simulink model "SinglePhaseControlledConveter"  (R2024a)
settings: Solver=VariableStepAuto  StartTime=0.0  StopTime=0.1  RelTol=1e-3
libraries: spsThyristorLib x4, spsCurrentMeasurementLib x2, spsVoltageMeasurementLib x2, spsACVoltageSourceLib x1, spsGroundLib x1, spsSeriesRLCBranchLib x1, spspowerguiLib x1
settings Model: Creator=danielmcguiness  LastModifiedBy=danielmcguiness

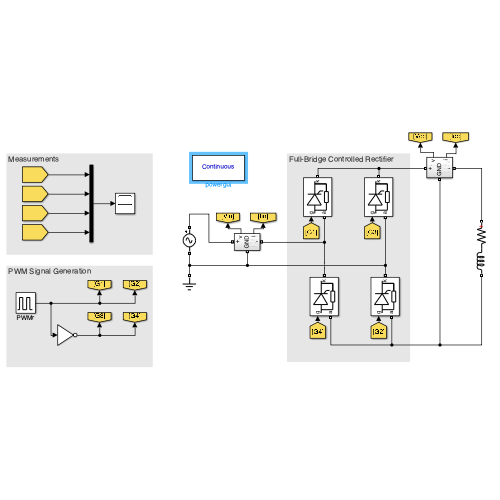
[thumbnail: Simulink's stored preview of the top-level diagram]
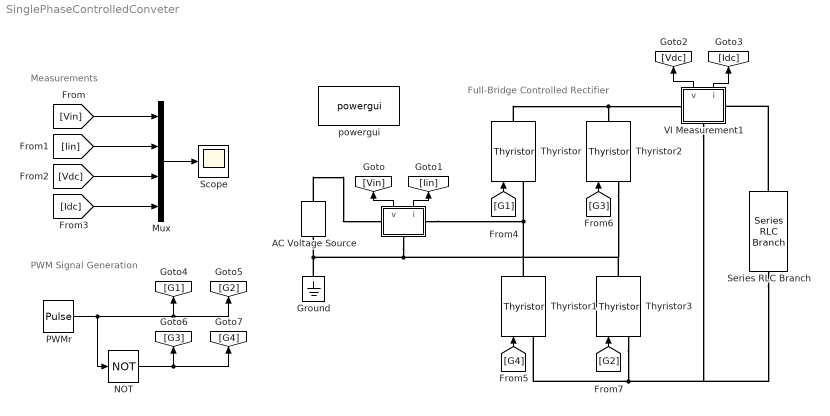
== system SinglePhaseControlledConveter ==
  note: PWM Signal Generation
  note: Measurements
  note: Full-Bridge Controlled Rectifier
  " " : Subsystem
      settings: PortSchema="{\"entries\":[{\"content\":{\"sides\":[{\"content\":{\"connectorIds\":[\"LConn1\"]},\"type\":\"ConnectorPlacement.EquallySpacedRectSide\",\"uuid\":\"19cbdb0e-db66-4f32-bba5-834b4ac7df8a\"},{\"content\":{\"connectorIds\":[\"RConn1\"],\"side\":\"RIGHT\"},\"type\":\"ConnectorPlacement.EquallySpacedRectSide\",\"uuid\":\"c14221e2-ec80-4808-9ed7-b609a9c8539a\"},{\"content\":{\"connectorIds\":[\"Out1\",\"Out2\"],\"side\":\"TOP\"},\"type\":\"ConnectorPlacement.EquallySpacedRectSide\",\"uuid\":\"b53df900-9b24-499c-9c1b-afbded56e9d5\"},{\"content\":{\"connectorIds\":[\"RConn2\"],\"side\":\"BOTTOM\"},\"type\":\"ConnectorPlacement.EquallySpacedRectSide\",\"uuid\":\"9b8e0864-8d67-4a67-b490-d2de7535cf50\"}]},\"type\":\"ConnectorPlacement.EquallySpacedConnector\",\"uuid\":\"ab9b4a2b-56b2-48b4-b21b-62113f75dc79\"}],\"packageUris\":[\"http://schema.mathworks.com/mf0/Connector/R2020b\"],\"version\":\"1.0\"}"
  AC Voltage Source : spsACVoltageSourceLib/AC Voltage Source  Amplitude=100  Phase=0  Frequency=50  SampleTime=0  Measurements=None  BusType=swing  Pref=10e3  Qref=0  Qmin=-inf  Qmax=+inf
  Ground : spsGroundLib/Ground  LConnTagsString=a
  Mux : Mux
  NOT : Logic  Operator=NOT  IconShape=distinctive  AllPortsSameDT=off  OutDataTypeStr=boolean
  PWMr : DiscretePulseGenerator  PulseType=Time based  Amplitude=100  Period=1/50  PulseWidth=50  PhaseDelay=(1/50) * (45/360)
  Scope : Scope
  Series RLC Branch : spsSeriesRLCBranchLib/Series RLC Branch  LConnTagsString=__new0  RConnTagsString=__new0  BranchType=RL  Resistance=1  Inductance=20e-3  SetiL0=off  InitialCurrent=0  Capacitance=1e-6  Setx0=off  InitialVoltage=0  Measurements=None
  Thyristor{,1..3} (4 alike) : spsThyristorLib/Thyristor  Ron=0.001  Lon=0  Vf=0.8  IC=0  Rs=500  Cs=250e-9  Measurements=off
  VI Measurement1 : Subsystem
      settings: PortSchema="{\"entries\":[{\"content\":{\"sides\":[{\"content\":{\"connectorIds\":[\"LConn1\"]},\"type\":\"ConnectorPlacement.EquallySpacedRectSide\",\"uuid\":\"d0d06b58-e7a6-4090-bc4f-be16d4258115\"},{\"content\":{\"connectorIds\":[\"RConn1\"],\"side\":\"RIGHT\"},\"type\":\"ConnectorPlacement.EquallySpacedRectSide\",\"uuid\":\"ec0e199e-bf94-46e5-8fb5-fcfe43c2f9e8\"},{\"content\":{\"connectorIds\":[\"Out1\",\"Out2\"],\"side\":\"TOP\"},\"type\":\"ConnectorPlacement.EquallySpacedRectSide\",\"uuid\":\"e633db83-a48d-4359-b0a8-630d80fecfae\"},{\"content\":{\"connectorIds\":[\"RConn2\"],\"side\":\"BOTTOM\"},\"type\":\"ConnectorPlacement.EquallySpacedRectSide\",\"uuid\":\"46b0a315-b5ae-4457-83c3-69b7a744a381\"}]},\"type\":\"ConnectorPlacement.EquallySpacedConnector\",\"uuid\":\"3aa23921-cdab-42f2-9dd1-6188dd33585f\"}],\"packageUris\":[\"http://schema.mathworks.com/mf0/Connector/R2020b\"],\"version\":\"1.0\"}"
  powergui : spspowerguiLib/powergui  Priority=1  SimulationMode=Continuous  SampleTime=50e-6  frequency=60  Iterations=50  frequencyindice=50  Pbase=100e6  ErrMax=1e-4  UnitsV=kV  UnitsW=MW  buscounter=0  FunctionMessages=off  echomessages=off  EnableUseOfTLC=off  CurrentSourceSwitches=off  DisableSnubberDevices=off  DisableRonSwitches=off  DisableVfSwitches=off  DisplayEquations=off  AutomaticDiscreteSolvers=off  SolverType=Tustin/Backward Euler (TBE)  Interpol=off  ExternalGateDelay=off  methode=off  Ts=100  x0status=blocks  SPID=on  SwTol=0  HookPort=off  NonlinearTolerance=1e-4  nMaxIteration=100  ContinueOnMaxIteration=off  RestoreLinks=warning  ResistiveCurrentMeasurement=off  Frange=[0:2:500]  Ylog=off  Xlog=on  ShowGrid=off  save=off  variable=ZData  structure=0  ZoomFFT=off  StartTime=0.0  cycles=1  DisplayStyle=1  fundamental=60  FreqAxis=off  MaxFrequency=1000  frequencyindicesteady=1  RmsSteady=1  display=off
  wires:
  " "/1(v) -> [Vin]
  " "/2(i) -> [Iin]
  Mux/1 -> Scope/1
  VI Measurement1/2(i) -> [Idc]
  VI Measurement1/1(v) -> [Vdc]
  [Vdc] -> Mux/3
  [G1] -> Thyristor/1
  [G4] -> Thyristor1/1
  [G3] -> Thyristor2/1
  [G2] -> Thyristor3/1
  PWMr/1 -> NOT/1, [G2], [G1]
  NOT/1 -> [G4], [G3]
  [Idc] -> Mux/4
  [Iin] -> Mux/2
  [Vin] -> Mux/1
  connections:
  Thyristor1/RConn1 -- " "/RConn1 -- Thyristor/LConn1
  Thyristor/RConn1 -- VI Measurement1/LConn1 -- Thyristor2/RConn1
  AC Voltage Source/RConn1 -- " "/LConn1
  Series RLC Branch/LConn1 -- VI Measurement1/RConn1
  Thyristor3/LConn1 -- VI Measurement1/RConn2 -- Series RLC Branch/RConn1 -- Thyristor1/LConn1
  " "/RConn2 -- Ground/LConn1 -- AC Voltage Source/LConn1 -- Thyristor2/LConn1 -- Thyristor3/RConn1

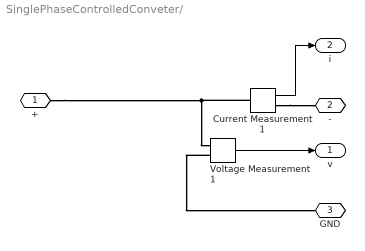
== system SinglePhaseControlledConveter/  ==
  Current Measurement1 : spsCurrentMeasurementLib/Current Measurement  PhasorSimulation=off  OutputType=Complex  PSBequivalent=0
  Voltage Measurement1 : spsVoltageMeasurementLib/Voltage Measurement  PhasorSimulation=off  OutputType=Complex  PSBequivalent=0
  + : PMIOPort  Side=Left
  - : PMIOPort  Port=2  Side=Right
  GND : PMIOPort  Port=3  Side=Right
  v : Outport
  i : Outport  Port=2
  wires:
  Voltage Measurement1/1 -> v/1
  Current Measurement1/1 -> i/1
  connections:
  Voltage Measurement1/LConn2 -- GND/RConn1
  Current Measurement1/RConn1 -- -/RConn1
  Current Measurement1/LConn1 -- Voltage Measurement1/LConn1 -- +/RConn1

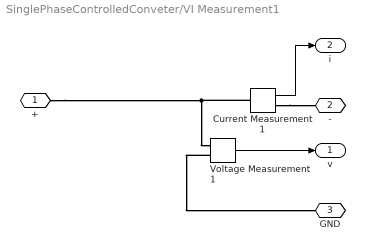
== system SinglePhaseControlledConveter/VI Measurement1 ==
  Current Measurement1 : spsCurrentMeasurementLib/Current Measurement  PhasorSimulation=off  OutputType=Complex  PSBequivalent=0
  Voltage Measurement1 : spsVoltageMeasurementLib/Voltage Measurement  PhasorSimulation=off  OutputType=Complex  PSBequivalent=0
  + : PMIOPort  Side=Left
  - : PMIOPort  Port=2  Side=Right
  GND : PMIOPort  Port=3  Side=Right
  v : Outport
  i : Outport  Port=2
  wires:
  Voltage Measurement1/1 -> v/1
  Current Measurement1/1 -> i/1
  connections:
  Current Measurement1/LConn1 -- Voltage Measurement1/LConn1 -- +/RConn1
  Voltage Measurement1/LConn2 -- GND/RConn1
  Current Measurement1/RConn1 -- -/RConn1
